simulink model "ImageAcquisitionAndColorSpaces"  (R2023a)
settings: Solver=ode4  StartTime=0.0  StopTime=inf  FixedStep=1/30  RelTol=1e-3  EnableMultiTasking=on
undefined symbols (not defined in the file): qc_get_step_size, Video3D
libraries: quarc_library x18
settings Model: SimulationMode=external  ExtModeTrigDuration=10000  Creator=fvranes  LastModifiedBy=mbohra
settings SolverCC: AlgebraicLoopSolver=TrustRegion  PositivePriorityOrder=on
settings DataIOCC: SaveOutput=off  SignalLogging=off  DSMLogging=off  SaveTime=off  ReturnWorkspaceOutputs=off
settings DebuggingCC: UnconnectedInputMsg=warning  UnconnectedOutputMsg=warning  UnconnectedLineMsg=warning  ArithmeticOperatorsInVariantConditions=warning
settings ModelReferenceCC: EnableRefExpFcnMdlSchedulingChecks=on
settings SFSimCC: SimUseLocalCustomCode=off  CustomCodeUndefinedFunction=UseInterfaceOnly
settings RTWCC: Description=QUARC Win64 Target Using Toolchain  SystemTargetFile=quarc_win64.tlc  TemplateMakefile=quarc_default_tmf  RTWUseLocalCustomCode=off  Toolchain=QUARC win64 | nmake (64-bit Windows)  BuildConfiguration=Faster Runs  DLArmComputeVersion=19.05
settings CodeAppCC: StateflowObjectComments=on
settings STFCustomTargetCC: SystemTargetFile=quarc_win64.tlc
settings GRTTargetCC: ParMdlRefBuildCompliant=off  CompOptLevelCompliant=off  CombineOutputUpdateFcns=off  MatFileLogging=off  CPPClassGenCompliant=off  GRTInterface=on  ExtMode=on  ExtModeMexFile=quarc_comm
settings ConfigComp: CovMetricSettings=dswe

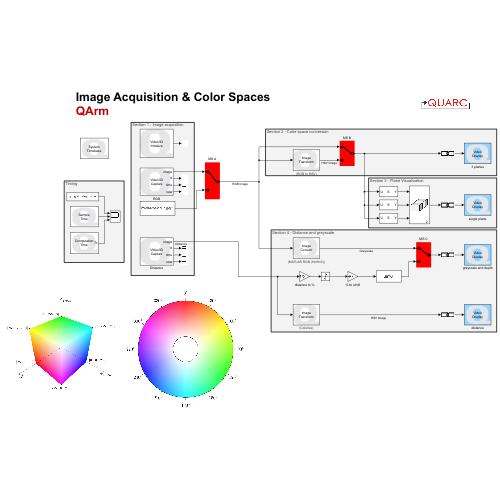
[thumbnail: Simulink's stored preview of the top-level diagram]
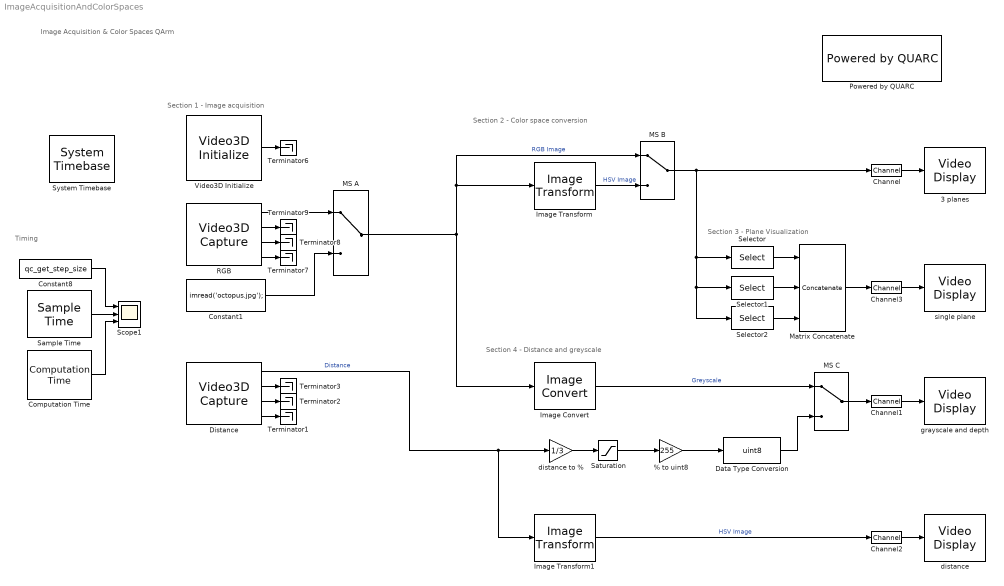
== system ImageAcquisitionAndColorSpaces ==
  note: Section 4 - Distance and greyscale
  note: Section 3 - Plane Visualization
  note: Section 2 - Color space conversion
  note: Timing
  note: Image Acquisition & Color Spaces
      | QArm
  note: Section 1 - Image acquisition
  % to uint8 : Gain  Gain=255
  3 planes : quarc_library/Multimedia/Video Display  Tag=ImageAcquisitionAndColorSpaces/3 planes  sample_time=-1  use_hardware=on
  Channel : quarc_library/Signal Routing/Channel  channel=0  buffer_size=1
  Channel1 : quarc_library/Signal Routing/Channel  channel=1  buffer_size=1
  Channel2 : quarc_library/Signal Routing/Channel  channel=2  buffer_size=1
  Channel3 : quarc_library/Signal Routing/Channel  channel=3  buffer_size=1
  Computation Time : quarc_library/Sources/Time/Computation Time  sample_time=qc_get_step_size  use_model=on  use_cpu_time=off
  Constant1 : Constant  Value=imread('octopus.jpg');
  Constant8 : Constant  Value=qc_get_step_size
  Data Type Conversion : DataTypeConversion  OutDataTypeStr=uint8  SaturateOnIntegerOverflow=off  RndMeth=Floor
  Distance : quarc_library/Multimedia/Video3D Capture  object_name=Video3D-1  stream_type=Depth  stream_index=0  resolution=640 x 480  width=640  height=480  output_format=Distance in meters (HxW)  data_type=single  sample_time=qc_get_step_size  camera_intrinsics=off  depth_scale=off  brightness_override=off  brightness=50.0  contrast_override=off  contrast=50.0  hue_override=off  hue=50.0  saturation_override=off  saturation=50.0  sharpness_override=off  sharpness=50.0  gamma_override=off  gamma=50.0  gain_override=off  gain=50.0  backlightcompensation_override=off  backlightcompensation=50.0  whitebalance_override=Automatic white balance  whitebalance=50.0  exposure_override=Automatic exposure  exposure=30.0  emitter=Enable laser emitter  preset=Do not set camera presets
  Image Convert : quarc_library/Image Processing/Generic/Image Convert  input_format=MATLAB RGB (HxWx3)  padding=0  output_format=MATLAB greyscale (HxW)  data_type=uint8
      settings: AttributesFormatString=(%<input_format>)  SourceProductName=QUARC Targets
  Image Transform : quarc_library/Image Processing/Generic/Image Transform  algorithm=RGB to HSV  color_theme=KRYGCBMW  min_pixel=0  max_pixel=4000  focal_length=308  principal_point=[262 334]  radial_coeffs=[-0.3129 0.0907]  tangential_coeffs=[]  extrapolated_pixel=0  interpolation=nearest  row_coords=0  column_coords=0  output_height=480  output_width=640  angle=0  origin=[240 320]  output_origin=[240 320]  output_data_type=uint8
      settings: AttributesFormatString=(%<algorithm>)  SourceProductName=QUARC Targets
  Image Transform1 : quarc_library/Image Processing/Generic/Image Transform  algorithm=Colorize  color_theme=KRYGCBMW  min_pixel=.2  max_pixel=3  focal_length=308  principal_point=[262 334]  radial_coeffs=[-0.3129 0.0907]  tangential_coeffs=[]  extrapolated_pixel=0  interpolation=nearest  row_coords=0  column_coords=0  output_height=480  output_width=640  angle=0  origin=[240 320]  output_origin=[240 320]  output_data_type=uint8
      settings: AttributesFormatString=(%<algorithm>)  SourceProductName=QUARC Targets
  MS A : ManualSwitch
  MS B : ManualSwitch
  MS C : ManualSwitch
  Matrix Concatenate : Concatenate  NumInputs=3  Mode=Multidimensional array  ConcatenateDimension=2
  Powered by QUARC : quarc_library/Logos/Powered by QUARC
  RGB : quarc_library/Multimedia/Video3D Capture  object_name=Video3D-1  stream_type=RGB  stream_index=0  resolution=640 x 480  width=640  height=480  output_format=MATLAB RGB (HxWx3)  data_type=uint8  sample_time=qc_get_step_size  camera_intrinsics=off  depth_scale=off  brightness_override=off  brightness=50.0  contrast_override=off  contrast=50.0  hue_override=off  hue=50.0  saturation_override=off  saturation=50.0  sharpness_override=off  sharpness=50.0  gamma_override=off  gamma=50.0  gain_override=off  gain=50.0  backlightcompensation_override=off  backlightcompensation=50.0  whitebalance_override=Automatic white balance  whitebalance=50.0  exposure_override=Automatic exposure  exposure=30.0  emitter=Enable laser emitter  preset=Do not set camera presets
  Sample Time : quarc_library/Sources/Time/Sample Time  Priority=-99  sample_time=qc_get_step_size
  Saturation : Saturate  UpperLimit=1  LowerLimit=0
  Scope1 : Scope  NumInputPorts=3
  Selector : Selector  NumberOfDimensions=3  InputPortWidth=3  IndexOptions=Select all,Select all,Index vector (dialog)  Indices=[1 3],1,1  OutputSizes=1,1,1
  Selector1 : Selector  NumberOfDimensions=3  InputPortWidth=3  IndexOptions=Select all,Select all,Index vector (dialog)  Indices=[1 3],1,2  OutputSizes=1,1,1
  Selector2 : Selector  NumberOfDimensions=3  InputPortWidth=3  IndexOptions=Select all,Select all,Index vector (dialog)  Indices=[1 3],1,3  OutputSizes=1,1,1
  System Timebase : quarc_library/Advanced/Timing/System Timebase  stop_on_overrun=off
      settings: SourceProductName=QUARC Targets
  Terminator{1..3,6..9} (7 alike) : Terminator
  Video3D Initialize : quarc_library/Multimedia/Video3D Initialize  object_name=Video3D-1  source=Device  identifier=0  file=sample.bag  sample_time=qc_get_step_size  active=on
  distance : quarc_library/Multimedia/Video Display  Tag=ImageAcquisitionAndColorSpaces/distance  sample_time=-1  use_hardware=on
  distance to % : Gain  Gain=1/3
  grayscale and depth : quarc_library/Multimedia/Video Display  Tag=ImageAcquisitionAndColorSpaces/grayscale and depth  sample_time=-1  use_hardware=on
  single plane : quarc_library/Multimedia/Video Display  Tag=ImageAcquisitionAndColorSpaces/single plane  sample_time=-1  use_hardware=on
  wires:
  RGB/3 -> Terminator8/1
  Video3D Initialize/1 -> Terminator6/1
  RGB/4 -> Terminator7/1
  RGB/2 -> Terminator9/1
  Sample Time/1 -> Scope1/2
  Constant8/1 -> Scope1/1
  Computation Time/1 -> Scope1/3
  Channel/1 -> 3 planes/1
  Distance/2 -> Terminator3/1
  Distance/3 -> Terminator2/1
  Distance/4 -> Terminator1/1
  Distance/1 -> Image Transform1/1, distance to %/1  "Distance"
  Channel1/1 -> grayscale and depth/1
  Channel2/1 -> distance/1
  Image Transform/1 -> MS B/2  "HSV Image"
  Image Transform1/1 -> Channel2/1  "HSV Image"
  MS A/1 -> MS B/1, Image Transform/1, Image Convert/1  "RGB Image"
  Image Convert/1 -> MS C/1  "Greyscale"
  MS B/1 -> Channel/1, Selector/1, Selector1/1, Selector2/1
  MS C/1 -> Channel1/1
  RGB/1 -> MS A/1
  distance to %/1 -> Saturation/1
  Channel3/1 -> single plane/1
  Selector/1 -> Matrix Concatenate/1
  Selector1/1 -> Matrix Concatenate/2
  Selector2/1 -> Matrix Concatenate/3
  Matrix Concatenate/1 -> Channel3/1
  Data Type Conversion/1 -> MS C/2
  % to uint8/1 -> Data Type Conversion/1
  Saturation/1 -> % to uint8/1
  Constant1/1 -> MS A/2
